simulink model "PMSM_HF_1_2019b"  (R2019b)
settings: Solver=ode4  StartTime=0.0  StopTime=4  FixedStep=Ts_model  RelTol=1e-3  EnableMultiTasking=on
InitFcn:
  | script_initfun;
undefined symbols (not defined in the file or in its folder): F, J, Ld, Lq, p, poles, R, Ts_model, Ts_torqueloop, Udc
libraries: powerlib x6, dsparch4 x4, simulink x3
settings Model: Creator=lovejing  LastModifiedBy=Administrator
settings SolverCC: ZeroCrossAlgorithm=Adaptive
settings DataIOCC: LimitDataPoints=on  SaveFormat=Array  ReturnWorkspaceOutputs=off
settings OptimizationCC: ExpressionDepthLimit=2147483647  LifeSpan=inf
settings DebuggingCC: UnderspecifiedInitializationDetection=Classic  MergeDetectMultiDrivingBlocksExec=none  SolverPrmCheckMsg=warning  FcnCallInpInsideContextMsg=warning  StateNameClashWarn=warning  SFUnexpectedBacktrackingDiag=warning  SFNoUnconditionalDefaultTransitionDiag=warning  SFExecutionAtInitializationDiag=none  ArithmeticOperatorsInVariantConditions=warning
settings HardwareCC: ProdBitPerPointer=32  ProdBitPerSizeT=32  ProdBitPerPtrDiffT=32  ProdLargestAtomicFloat=None  ProdIntDivRoundTo=Undefined  ProdEndianess=Unspecified  ProdWordSize=32  ProdHWDeviceType=32-bit Generic
settings ModelReferenceCC: PropagateSignalLabelsOutOfModel=off
settings SFSimCC: SimUseLocalCustomCode=off  CustomCodeUndefinedFunction=UseInterfaceOnly
settings RTWCC: RTWUseLocalCustomCode=off
settings CodeAppCC: StateflowObjectComments=on
settings GRTTargetCC: TargetLangStandard=C89/C90 (ANSI)  CombineOutputUpdateFcns=off  GRTInterface=on
settings ConfigComp: CovMetricSettings=dw  CovHtmlReporting=on  CovSaveCumulativeToWorkspaceVar=on  CovSaveSingleToWorkspaceVar=on  CovExternalEMLEnable=off  CovSFcnEnable=off
settings SimscapeCC: SimscapeNormalizeSystem=off

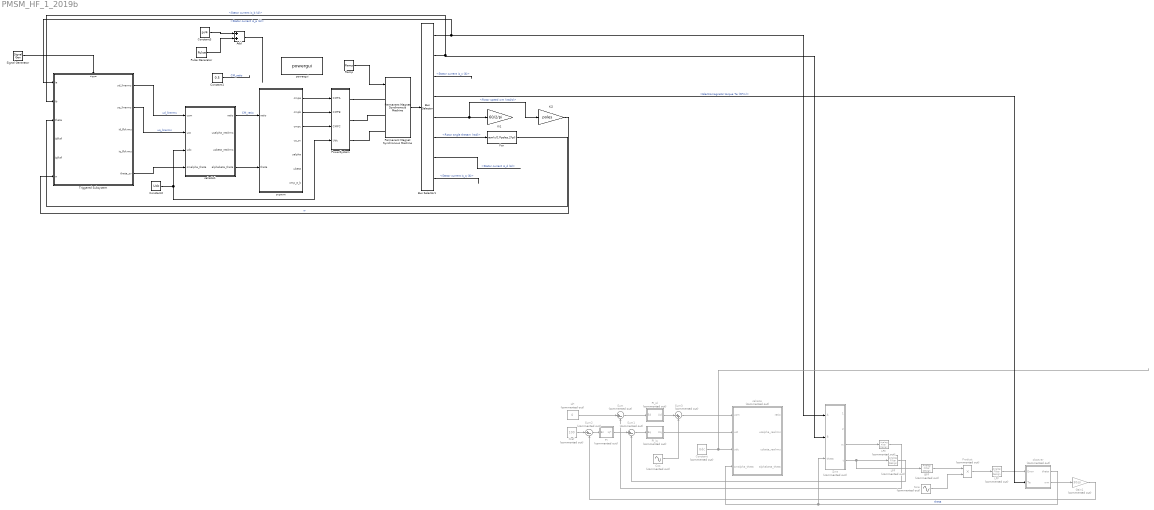
== system PMSM_HF_1_2019b ==
  " LPF" : dsparch4/Analog Filter Design  Commented=on  method=Butterworth  filttype=Lowpass  N=1  Wlo=942  Whi=80  Rp=2  Rs=40
  Add : Sum
  BPF : dsparch4/Analog Filter Design  Commented=on  method=Butterworth  filttype=Bandpass  N=2  Wlo=6200  Whi=6360  Rp=2  Rs=40
  Bus Selector1 : BusSelector  OutputSignals=Stator current is_a (A),Stator current is_b (A),Stator current is_c (A),Electromagnetic torque Te (N*m),Rotor speed wm (rad/s),Rotor angle thetam (rad),Stator current is_d (A),Stator current is_q (A)
  Constant : Constant  Commented=on  Value=Udc
  Constant1 : Constant  Value=0.5
  Constant2 : Constant  Value=Udc
  Constant3 : Constant  Value=pi/4
  Cos : Sin  Commented=on  Amplitude=20  Frequency=6280  Phase=pi/2  SampleTime=0
  Fcn : Fcn  Expr=rem(u(1)*poles,2*pi)
  Gain1 : Gain  Commented=on  Gain=30/pi
  Ki1 : Gain  Gain=60/2/pi
  Ki2 : Gain  Gain=poles
  LPF : dsparch4/Analog Filter Design  Commented=on  method=Butterworth  filttype=Lowpass  N=1  Wlo=942  Whi=80  Rp=2  Rs=40
  "LPF " : dsparch4/Analog Filter Design  Commented=on  method=Butterworth  filttype=Lowpass  N=1  Wlo=942  Whi=80  Rp=2  Rs=40
  Nref : Constant  Commented=on  Value=100
  PI : Subsystem  Commented=on  mask{Knp=0.4, Kni=2}
  PI_id : Subsystem  Commented=on  mask{Kip=40, Kii=1}
  PI_iq : Subsystem  Commented=on  mask{Kip=40, Kii=1}
  Permanent Magnet Synchronous Machine : powerlib/Machines/Permanent Magnet Synchronous Machine  NbPhases=3  FluxDistribution=Sinusoidal  RotorType=Salient-pole  MechanicalLoad=Speed w  PresetModel=No  ShowDetailedParameters=on  MeasurementBus=off  Resistance=R  Inductance=8.5e-3  dqInductances=[Ld Lq]  La=0.000835  MachineConstant=Torque Constant (N.m / A_peak)  Flux=0.085714  VoltageCst=62.1874  TorqueCst=180/350  Flat=120  Mechanical=[J F p 0]  PolePairs=poles  InitialConditions=[0,0, 0,0]  InitialConditions5ph=[0 0 0 0 0 0]  RefAngle=Aligned with phase A axis (original Park)  IterativeDiscreteModel=Trapezoidal non iterative  TsBlock=-1  TsPowergui=0
  PowerSystem : Subsystem
  Product : Product  Commented=on
  Pulse Generator : DiscretePulseGenerator  PulseType=Time based  Amplitude=pi  Period=0.001  PulseWidth=50
  Ramp : simulink/Sources/Ramp  slope=1  start=9  InitialOutput=0
  Signal Generator : SignalGenerator  WaveForm=square  Frequency=1/Ts_torqueloop
      settings: AttributesFormatString=Waveform: %<waveform>\nFreq: %<Frequency> %<Units>
  "Sine " : Sin  Commented=on  Frequency=6280  SampleTime=0
  Sum : Sum  Commented=on  Inputs=|+-
  Sum1 : Sum  Commented=on  Inputs=|+-
  Sum2 : Sum  Commented=on  Inputs=|+-
  Sum3 : Sum  Commented=on  Inputs=|++
  Triggered Subsystem : Subsystem  TreatAsAtomicUnit=on
  calratio : MATLAB Function  Commented=on  TreatAsAtomicUnit=on
  calratio1 : MATLAB Function  TreatAsAtomicUnit=on
  i2mt : MATLAB Function  Commented=on  TreatAsAtomicUnit=on
  id* : Constant  Commented=on  Value=0
  obsever : Subsystem  Commented=on
  powergui : powerlib/powergui  Priority=1  SimulationMode=Discrete  SampleTime=Ts_model  frequency=60  Iterations=50  frequencyindice=0  Pbase=100e6  ErrMax=1e-4  UnitsV=kV  UnitsW=MW  buscounter=0  FunctionMessages=off  echomessages=off  EnableUseOfTLC=off  CurrentSourceSwitches=off  DisableSnubberDevices=off  DisableRonSwitches=off  DisableVfSwitches=off  DisplayEquations=off  AutomaticDiscreteSolvers=off  SolverType=Tustin/Backward Euler (TBE)  Interpol=off  ExternalGateDelay=off  methode=off  Ts=100  x0status=blocks  SPID=on  SwTol=0  HookPort=off  NonlinearTolerance=0  nMaxIteration=15  ContinueOnMaxIteration=off  RestoreLinks=warning  ResistiveCurrentMeasurement=off  Frange=[0:2:500]  Ylog=off  Xlog=on  ShowGrid=off  save=off  variable=ZData  structure=0  ZoomFFT=off  StartTime=0.0  cycles=1  DisplayStyle=1  fundamental=60  FreqAxis=off  MaxFrequency=1000  frequencyindicesteady=1  RmsSteady=1  display=off
      settings: SourceProductName=Simscape Electrical
  svpwm : MATLAB Function  TreatAsAtomicUnit=on
  wires:
  id*/1 -> Sum/1
  LPF/1 -> Sum/2
  Sum/1 -> PI_id/1(Ed)
  "LPF "/1 -> Sum1/2
  Nref/1 -> Sum2/1
  Sum2/1 -> PI/1(En)
  Sum1/1 -> PI_iq/1(Eq)
  PI/1(iq*) -> Sum1/1
  PI_iq/1(Uq) -> calratio/2(ust)
  obsever/2(wm) -> Gain1/1
  Product/1 -> " LPF"/1
  Sum3/1 -> calratio/1(usm)
  PI_id/1(Ud) -> Sum3/1
  Cos/1 -> Sum3/2
  i2mt/3(m) -> LPF/1
  i2mt/4(t) -> BPF/1, "LPF "/1
  BPF/1 -> Product/1
  "Sine "/1 -> Product/2
  Gain1/1 -> Sum2/2
  obsever/1(theta) -> i2mt/3(theta), calratio/4(smalpha_theta)  "theta"
  " LPF"/1 -> obsever/1(Error)
  svpwm/2(cmpb) -> PowerSystem/2(CMPB)
  svpwm/3(cmpc) -> PowerSystem/3(CMPC)
  Constant1/1 -> ?  "CM_ratio"
  svpwm/1(cmpa) -> PowerSystem/1(CMPA)
  Add/1 -> ?
  Bus Selector1/6 -> Fcn/1  "<Rotor angle thetam (rad)>"
  Permanent Magnet Synchronous Machine/1 -> Bus Selector1/1
  Ramp/1 -> Permanent Magnet Synchronous Machine/1
  Bus Selector1/1 -> i2mt/1(A), Triggered Subsystem/1(ia)  "<Stator current is_a (A)>"
  Bus Selector1/2 -> Triggered Subsystem/2(ib), i2mt/2(B)  "<Stator current is_b (A)>"
  Constant/1 -> calratio/3(udc)
  Bus Selector1/7 -> ?  "<Stator current is_d (A)>"
  Bus Selector1/8 -> ?  "<Stator current is_q (A)>"
  Bus Selector1/4 -> obsever/2(Te)  "<Electromagnetic torque Te (N*m)>"
  Bus Selector1/3 -> ?  "<Stator current is_c (A)>"
  Constant3/1 -> Add/1
  Pulse Generator/1 -> Add/2
  Signal Generator/1 -> Triggered Subsystem/Trigger
  Triggered Subsystem/1(ud_linerms) -> calratio1/1(usm)  "ud_linerms"
  Triggered Subsystem/2(uq_linerms) -> calratio1/2(ust)  "uq_linerms"
  Constant2/1 -> PowerSystem/4(Udc), calratio1/3(udc)
  Triggered Subsystem/5(theta_sv) -> calratio1/4(smalpha_theta)
  calratio1/1(ratio) -> svpwm/1(ratio)  "CM_ratio"
  calratio1/4(alphabeta_theta) -> svpwm/2(theta)
  Fcn/1 -> Triggered Subsystem/3(theta)
  Bus Selector1/5 -> Ki2/1, Ki1/1  "<Rotor speed wm (rad/s)>"
  Ki2/1 -> Triggered Subsystem/6(w)  "w"
  connections:
  PowerSystem/RConn1 -- Permanent Magnet Synchronous Machine/LConn1
  PowerSystem/RConn2 -- Permanent Magnet Synchronous Machine/LConn2
  PowerSystem/RConn3 -- Permanent Magnet Synchronous Machine/LConn3

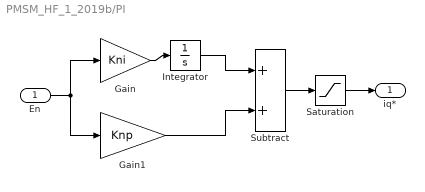
== system PMSM_HF_1_2019b/PI ==
  En : Inport
  Gain : Gain  Gain=Kni
  Gain1 : Gain  Gain=Knp
  Integrator : Integrator
  Saturation : Saturate  UpperLimit=50  LowerLimit=-50
  Subtract : Sum
  iq* : Outport
  wires:
  En/1 -> Gain/1, Gain1/1
  Gain/1 -> Integrator/1
  Integrator/1 -> Subtract/1
  Gain1/1 -> Subtract/2
  Subtract/1 -> Saturation/1
  Saturation/1 -> iq*/1

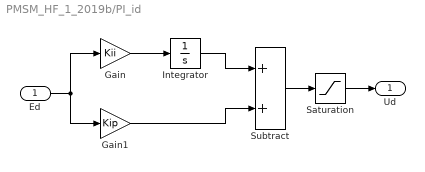
== system PMSM_HF_1_2019b/PI_id ==
  Ed : Inport
  Gain : Gain  Gain=Kii
  Gain1 : Gain  Gain=Kip
  Integrator : Integrator
  Saturation : Saturate  UpperLimit=10  LowerLimit=-10
  Subtract : Sum
  Ud : Outport
  wires:
  Ed/1 -> Gain/1, Gain1/1
  Gain/1 -> Integrator/1
  Integrator/1 -> Subtract/1
  Gain1/1 -> Subtract/2
  Subtract/1 -> Saturation/1
  Saturation/1 -> Ud/1

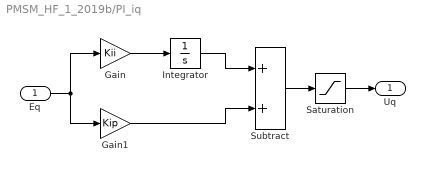
== system PMSM_HF_1_2019b/PI_iq ==
  Eq : Inport
  Gain : Gain  Gain=Kii
  Gain1 : Gain  Gain=Kip
  Integrator : Integrator
  Saturation : Saturate  UpperLimit=100  LowerLimit=-100
  Subtract : Sum
  Uq : Outport
  wires:
  Eq/1 -> Gain/1, Gain1/1
  Gain/1 -> Integrator/1
  Integrator/1 -> Subtract/1
  Gain1/1 -> Subtract/2
  Subtract/1 -> Saturation/1
  Saturation/1 -> Uq/1

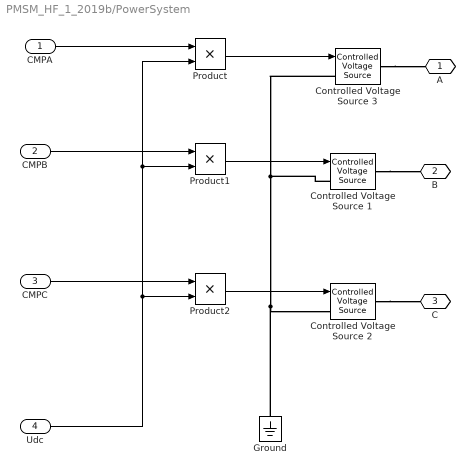
== system PMSM_HF_1_2019b/PowerSystem ==
  CMPA : Inport
  CMPB : Inport  Port=2
  CMPC : Inport  Port=3
  Udc : Inport  Port=4
  Controlled Voltage Source 1 : powerlib/Electrical Sources/Controlled Voltage Source  Initialize=on  Source_Type=AC  Amplitude=300  Phase=0  Frequency=0  Measurements=None
      settings: SourceProductName=Simscape Electrical
  Controlled Voltage Source 2 : powerlib/Electrical Sources/Controlled Voltage Source  Initialize=on  Source_Type=AC  Amplitude=300  Phase=0  Frequency=0  Measurements=None
      settings: SourceProductName=Simscape Electrical
  Controlled Voltage Source 3 : powerlib/Electrical Sources/Controlled Voltage Source  Initialize=on  Source_Type=AC  Amplitude=300  Phase=0  Frequency=0  Measurements=None
      settings: SourceProductName=Simscape Electrical
  Ground : powerlib/Elements/Ground  LConnTagsString=a
      settings: SourceProductName=Simscape Electrical
  Product : Product
  Product1 : Product
  Product2 : Product
  A : PMIOPort  Side=Right
  B : PMIOPort  Port=2  Side=Right
  C : PMIOPort  Port=3  Side=Right
  wires:
  Udc/1 -> Product2/2, Product1/2, Product/2
  Product2/1 -> Controlled Voltage Source 2/1
  Product1/1 -> Controlled Voltage Source 1/1
  Product/1 -> Controlled Voltage Source 3/1
  CMPA/1 -> Product/1
  CMPB/1 -> Product1/1
  CMPC/1 -> Product2/1
  connections:
  Controlled Voltage Source 1/LConn1 -- Controlled Voltage Source 3/LConn1 -- Ground/LConn1 -- Controlled Voltage Source 2/LConn1
  Controlled Voltage Source 3/RConn1 -- A/RConn1
  Controlled Voltage Source 1/RConn1 -- B/RConn1
  Controlled Voltage Source 2/RConn1 -- C/RConn1

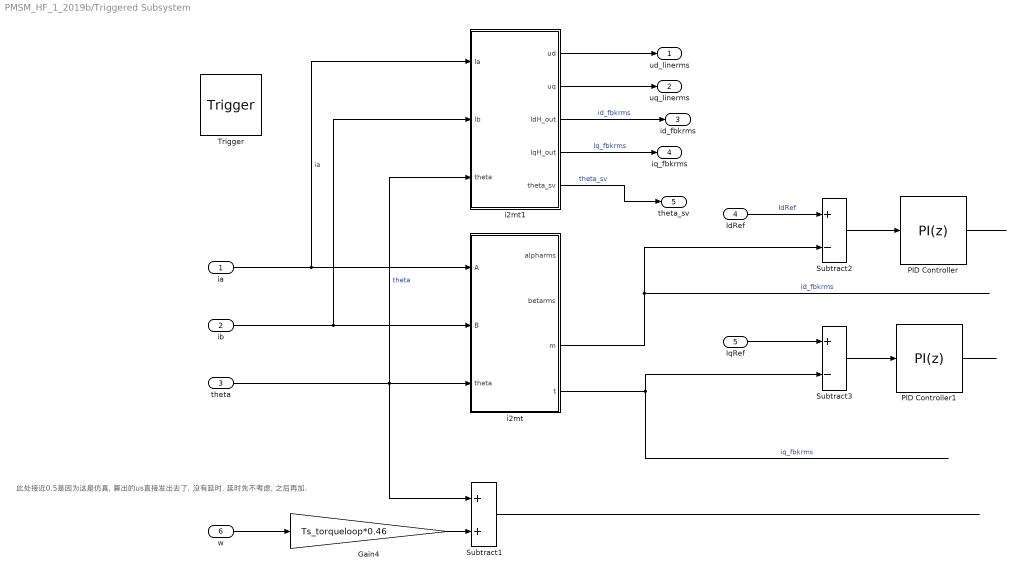
== system PMSM_HF_1_2019b/Triggered Subsystem ==
  note: 此处接近0.5是因为这是仿真, 算出的us直接发出去了, 没有延时. 延时先不考虑, 之后再加.
  ia : Inport
  ib : Inport  Port=2
  theta : Inport  Port=3
  IdRef : Inport  Port=4
  IqRef : Inport  Port=5
  w : Inport  Port=6
  Trigger : TriggerPort  VariantControl=(inherit)
  Gain4 : Gain  Gain=Ts_torqueloop*0.46
  PID Controller : simulink/Continuous/PID Controller  Controller=PI  Form=Parallel  TimeDomain=Discrete-time  SampleTime=-1  IntegratorMethod=Trapezoidal  FilterMethod=Forward Euler  ControllerParametersSource=internal  P=4  I=100  D=0  UseFilter=on  N=100  TunerSelectOption=Transfer Function Based (PID Tuner App)  InitialConditionSource=internal  InitialConditionForIntegrator=0  InitialConditionForFilter=0  DifferentiatorICPrevScaledInput=0  ExternalReset=none  TrackingMode=off  Kt=1  LimitOutput=on  UpperSaturationLimit=Udc/sqrt(2)*1.1  LowerSaturationLimit=-Udc/sqrt(2)*1.1  LinearizeAsGain=on  AntiWindupMode=none  Kb=1  POutMin=[]  POutMax=[]  IOutMin=[]  IOutMax=[]  DOutMin=[]  DOutMax=[]  NOutMin=[]  NOutMax=[]  SumOutMin=[]  SumOutMax=[]  SaturationOutMin=[]  SaturationOutMax=[]  PParamMin=[]  PParamMax=[]  IParamMin=[]  IParamMax=[]  DParamMin=[]  DParamMax=[]  NParamMin=[]  NParamMax=[]  KbParamMin=[]  KbParamMax=[]  KtParamMin=[]  KtParamMax=[]  KbOutMin=[]  KbOutMax=[]  KtOutMin=[]  KtOutMax=[]  IntegratorOutMin=[]  IntegratorOutMax=[]  FilterOutMin=[]  FilterOutMax=[]  SumI1OutMin=[]  SumI1OutMax=[]  SumI2OutMin=[]  SumI2OutMax=[]  SumI3OutMin=[]  SumI3OutMax=[]  SumI4OutMin=[]  SumI4OutMax=[]  SumDOutMin=[]  SumDOutMax=[]  DifferentiatorOutMin=[]  DifferentiatorOutMax=[]  FilterDiffOutCoefMin=[]  FilterDiffOutCoefMax=[]  ReciprocalOutMin=[]  ReciprocalOutMax=[]  SumDenOutMin=[]  SumDenOutMax=[]  SumNumOutMin=[]  SumNumOutMax=[]  DivideOutMin=[]  DivideOutMax=[]  IntegratorContinuousStateAttributes=''  IntegratorStateMustResolveToSignalObject=off  IntegratorRTWStateStorageClass=Auto  FilterContinuousStateAttributes=''  FilterStateMustResolveToSignalObject=off  FilterRTWStateStorageClass=Auto  ParallelPVariant=InternalParameters  IdealPVariant=Disabled  IVariant=InternalParameters  DVariant=Disabled  IntegratorVariant=Discrete  SatVariant=Enabled  AWVariant=Passthrough  PCopyVariant=Disabled  TRVariant=Disabled  FdbkBlocksVariant=Forward  IdealPFdbkVariant=Disabled  SatFdbkVariant=Disabled  DerivativeFilterVariant=Disabled  NVariant=Disabled  NCopyVariant=Disabled_SignalSpec  FilterICVariant=Disabled  IntegratorICVariant=InternalICs  ExternalResetVariant=Disabled  TRSumVariant=Passthrough  SumFdbkVariant=Disabled  SumVariant=Sum_PI
  PID Controller1 : simulink/Continuous/PID Controller  Controller=PI  Form=Parallel  TimeDomain=Discrete-time  SampleTime=-1  IntegratorMethod=Trapezoidal  FilterMethod=Forward Euler  ControllerParametersSource=internal  P=4  I=100  D=0  UseFilter=on  N=100  TunerSelectOption=Transfer Function Based (PID Tuner App)  InitialConditionSource=internal  InitialConditionForIntegrator=0  InitialConditionForFilter=0  DifferentiatorICPrevScaledInput=0  ExternalReset=none  TrackingMode=off  Kt=1  LimitOutput=on  UpperSaturationLimit=Udc/sqrt(2)*1.1  LowerSaturationLimit=-Udc/sqrt(2)*1.1  LinearizeAsGain=on  AntiWindupMode=none  Kb=1  POutMin=[]  POutMax=[]  IOutMin=[]  IOutMax=[]  DOutMin=[]  DOutMax=[]  NOutMin=[]  NOutMax=[]  SumOutMin=[]  SumOutMax=[]  SaturationOutMin=[]  SaturationOutMax=[]  PParamMin=[]  PParamMax=[]  IParamMin=[]  IParamMax=[]  DParamMin=[]  DParamMax=[]  NParamMin=[]  NParamMax=[]  KbParamMin=[]  KbParamMax=[]  KtParamMin=[]  KtParamMax=[]  KbOutMin=[]  KbOutMax=[]  KtOutMin=[]  KtOutMax=[]  IntegratorOutMin=[]  IntegratorOutMax=[]  FilterOutMin=[]  FilterOutMax=[]  SumI1OutMin=[]  SumI1OutMax=[]  SumI2OutMin=[]  SumI2OutMax=[]  SumI3OutMin=[]  SumI3OutMax=[]  SumI4OutMin=[]  SumI4OutMax=[]  SumDOutMin=[]  SumDOutMax=[]  DifferentiatorOutMin=[]  DifferentiatorOutMax=[]  FilterDiffOutCoefMin=[]  FilterDiffOutCoefMax=[]  ReciprocalOutMin=[]  ReciprocalOutMax=[]  SumDenOutMin=[]  SumDenOutMax=[]  SumNumOutMin=[]  SumNumOutMax=[]  DivideOutMin=[]  DivideOutMax=[]  IntegratorContinuousStateAttributes=''  IntegratorStateMustResolveToSignalObject=off  IntegratorRTWStateStorageClass=Auto  FilterContinuousStateAttributes=''  FilterStateMustResolveToSignalObject=off  FilterRTWStateStorageClass=Auto  ParallelPVariant=InternalParameters  IdealPVariant=Disabled  IVariant=InternalParameters  DVariant=Disabled  IntegratorVariant=Discrete  SatVariant=Enabled  AWVariant=Passthrough  PCopyVariant=Disabled  TRVariant=Disabled  FdbkBlocksVariant=Forward  IdealPFdbkVariant=Disabled  SatFdbkVariant=Disabled  DerivativeFilterVariant=Disabled  NVariant=Disabled  NCopyVariant=Disabled_SignalSpec  FilterICVariant=Disabled  IntegratorICVariant=InternalICs  ExternalResetVariant=Disabled  TRSumVariant=Passthrough  SumFdbkVariant=Disabled  SumVariant=Sum_PI
  Subtract1 : Sum
  Subtract2 : Sum  Inputs=+-
  Subtract3 : Sum  Inputs=+-
  i2mt : MATLAB Function  TreatAsAtomicUnit=on
  i2mt1 : MATLAB Function  TreatAsAtomicUnit=on
  ud_linerms : Outport
  uq_linerms : Outport  Port=2
  id_fbkrms : Outport  Port=3
  iq_fbkrms : Outport  Port=4
  theta_sv : Outport  Port=5
  wires:
  Subtract1/1 -> ?
  Gain4/1 -> Subtract1/2
  theta/1 -> i2mt1/3(theta), i2mt/3(theta), Subtract1/1  "theta"
  ib/1 -> i2mt1/2(Ib), i2mt/2(B)
  i2mt/4(t) -> Subtract3/2  "iq_fbkrms"
  i2mt/3(m) -> Subtract2/2  "id_fbkrms"
  w/1 -> Gain4/1
  ia/1 -> i2mt1/1(Ia), i2mt/1(A)  "ia"
  Subtract2/1 -> PID Controller/1
  PID Controller/1 -> ?
  IdRef/1 -> Subtract2/1  "IdRef"
  IqRef/1 -> Subtract3/1
  Subtract3/1 -> PID Controller1/1
  PID Controller1/1 -> ?
  i2mt1/1(ud) -> ud_linerms/1
  i2mt1/2(uq) -> uq_linerms/1
  i2mt1/5(theta_sv) -> theta_sv/1  "theta_sv"
  i2mt1/4(IqH_out) -> iq_fbkrms/1  "Iq_fbkrms"
  i2mt1/3(IdH_out) -> id_fbkrms/1  "id_fbkrms"

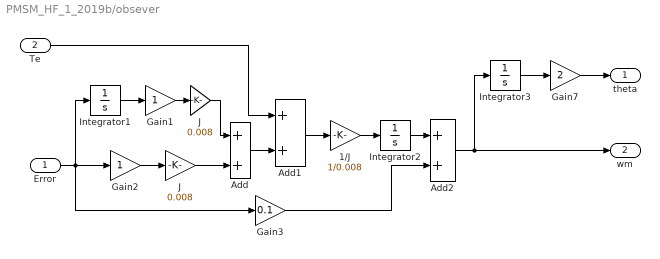
== system PMSM_HF_1_2019b/obsever ==
  Error : Inport
  Te : Inport  Port=2
  1/J : Gain  Gain=1/0.008
  Add : Sum
  Add1 : Sum
  Add2 : Sum
  Gain1 : Gain
  Gain2 : Gain
  Gain3 : Gain  Gain=0.1
  Gain7 : Gain  Gain=2
  Integrator1 : Integrator
  Integrator2 : Integrator
  Integrator3 : Integrator
  J : Gain  Gain=0.008
  "J " : Gain  Gain=0.008
  theta : Outport
  wm : Outport  Port=2
  wires:
  Error/1 -> Integrator1/1, Gain2/1, Gain3/1
  Integrator1/1 -> Gain1/1
  Add/1 -> Add1/2
  1/J/1 -> Integrator2/1
  Integrator2/1 -> Add2/1
  Add2/1 -> Integrator3/1, wm/1
  Gain2/1 -> "J "/1
  Gain1/1 -> J/1
  Gain3/1 -> Add2/2
  Integrator3/1 -> Gain7/1
  Add1/1 -> 1/J/1
  Te/1 -> Add1/1
  Gain7/1 -> theta/1
  J/1 -> Add/1
  "J "/1 -> Add/2

== matlab function PMSM_HF_1_2019b/svpwm ==
  data: cmpa output; cmpb output; cmpc output; us_sv output; ualpha output; ubeta output; ratio input; cmp_a_b output; theta input
%% intro
% u1: ratio, 0~1.155
% u2: theta, -pi~pi,
% us_sv: us in sv

%% function
function [cmpa, cmpb, cmpc, us_sv, ualpha, ubeta, cmp_a_b] = svpwm(ratio, theta)

[cmpa, cmpb, cmpc, us_sv, ualpha, ubeta, cmp_a_b] = script_svpwm(ratio, theta);

== matlab function PMSM_HF_1_2019b/Triggered Subsystem/i2mt ==
  data: alpharms output; betarms output; A input; m output; B input; theta input; t output
function [alpharms, betarms, m, t] = fcn(A, B, theta)
Arms = A/sqrt(2);
Brms = B/sqrt(2);

alpharms = Arms;
betarms = (Arms + 2*Brms)*sqrt(3)/3;


[m, t] = script_qd2mt(alpharms, betarms, theta);

== matlab function PMSM_HF_1_2019b/calratio1 ==
  data: ratio output; usm input; ust input; udc input; usalpha_realrms output; usbeta_realrms output; alphabeta_theta output; smalpha_theta input
%% intro
% u1: ratio, 0~1.155
% u2: theta, -pi~pi,
% us_sv: us in sv

%% function
function [ratio, usalpha_realrms, usbeta_realrms, alphabeta_theta]  = calratio(usm, ust, udc, smalpha_theta)

ualpha = - ust*sin(smalpha_theta) + usm*cos(smalpha_theta);
ubeta = usm*sin(smalpha_theta) + ust*cos(smalpha_theta);


alphabeta_theta = atan2(ubeta, ualpha);

us2 = ualpha*ualpha + ubeta*ubeta;  % rms
us = sqrt(us2);
if us > udc*1.103/sqrt(2)
    us = udc*1.103/sqrt(2);
end
usalpha_realrms = us * cos(alphabeta_theta);
usbeta_realrms = us * sin(alphabeta_theta);

ratio = us*sqrt(2)/udc;

== matlab function PMSM_HF_1_2019b/calratio ==
  data: ratio output; usm input; ust input; udc input; usalpha_realrms output; usbeta_realrms output; alphabeta_theta output; smalpha_theta input
%% intro
% u1: ratio, 0~1.155
% u2: theta, -pi~pi,
% us_sv: us in sv

%% function
function [ratio, usalpha_realrms, usbeta_realrms, alphabeta_theta]  = calratio(usm, ust, udc, smalpha_theta)

ualpha = - ust*sin(smalpha_theta) + usm*cos(smalpha_theta);
ubeta = usm*sin(smalpha_theta) + ust*cos(smalpha_theta);


alphabeta_theta = atan2(ubeta, ualpha);

us2 = ualpha*ualpha + ubeta*ubeta;  % rms
us = sqrt(us2);
if us > udc*1.103/sqrt(2)
    us = udc*1.103/sqrt(2);
end
usalpha_realrms = us * cos(alphabeta_theta);
usbeta_realrms = us * sin(alphabeta_theta);

ratio = us*sqrt(2)/udc;

== matlab function PMSM_HF_1_2019b/i2mt ==
  data: alpharms output; betarms output; A input; m output; B input; theta input; t output
function [alpharms, betarms, m, t] = fcn(A, B, theta)
Arms = A/sqrt(2);
Brms = B/sqrt(2);

alpharms = Arms;
betarms = (Arms + 2*Brms)*sqrt(3)/3;


[m, t] = script_qd2mt(alpharms, betarms, theta);

== matlab function PMSM_HF_1_2019b/Triggered Subsystem/i2mt1 ==
  data: ud output; uq output; Ia input; IdH_out output; IqH_out output; Ib input; theta input; theta_sv output
function [ud, uq, IdH_out, IqH_out, theta_sv] = fcn(Ia, Ib, theta)

persistent cnt;if(isempty(cnt)),    cnt = 0;end
persistent IaHis;if(isempty(IaHis)),    IaHis = 0;end
persistent IbHis;if(isempty(IbHis)),    IbHis = 0;end
persistent Iadelta;if(isempty(Iadelta)),    Iadelta = 0;end
persistent Ibdelta;if(isempty(Ibdelta)),    Ibdelta = 0;end
persistent IdH;if(isempty(IdH)),    IdH = 0;end
persistent IqH; if(isempty(IqH)),    IqH = 0;    end
persistent testthetacnt; if(isempty(testthetacnt)),    testthetacnt = 0;    end
persistent theta_out; if(isempty(theta_out)),    theta_out = 1*pi/4;    end

% TrqLoop every 100us, 10times equal 2ms, 
cnt = cnt + 1;
% 1~20 output 100V, 21~40 output -100V
if(cnt <= 20)
    ud = 100; %100V
elseif(cnt < 40)
    ud = -100;
else
    ud = -100;
    cnt = 0;
end

uq = 0;
 theta_sv = theta + - pi/4;    % hfi in 45degree after d_axis.
% 
 testthetacnt = testthetacnt + 1;
 theta_sv = rem(testthetacnt/1000*pi, 2*pi);


% current
if(cnt == 1)    % last point of -100V
    Iadelta = Ia - IaHis;
    Ibdelta = Ib - IbHis;
    IaHis = Ia;
    IbHis = Ib;
    
    Arms = Iadelta/sqrt(2);
    Brms = Ibdelta/sqrt(2);
    alpharms = Arms;
    betarms = (Arms + 2*Brms)*sqrt(3)/3;
    [IdH, IqH] = script_qd2mt(alpharms, betarms, theta_sv + pi);
   % theta_out = theta_out + (IqH)*0.001;
elseif(cnt == 21)   % last point of 100V
    Iadelta = Ia - IaHis;
    Ibdelta = Ib - IbHis;
    IaHis = Ia;
    IbHis = Ib;
    
    Arms = Iadelta/sqrt(2);
    Brms = Ibdelta/sqrt(2);
    alpharms = Arms;
    betarms = (Arms + 2*Brms)*sqrt(3)/3;
    [IdH, IqH] = script_qd2mt(alpharms, betarms, theta_sv);
   % theta_out = theta_out + (IqH)*0.001;
end


%theta_sv = rem(theta_out, 2*pi);




IdH_out = IdH;
IqH_out = IqH;
